simulink model "IGRF_Model"  (R2024a)
settings: Solver=VariableStepAuto  StartTime=0.0  StopTime=10.0  RelTol=1e-3
undefined symbols (not defined in the file or in its folder): WMM2020
libraries: sharedtransform x1, aerolibgravity2 x1
settings Model: Creator=hendr  LastModifiedBy=hendr

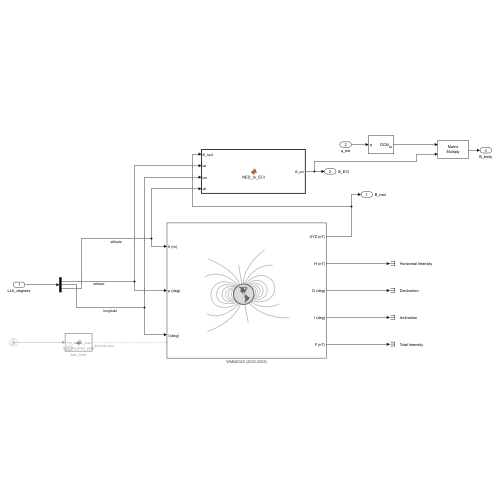
[thumbnail: Simulink's stored preview of the top-level diagram]
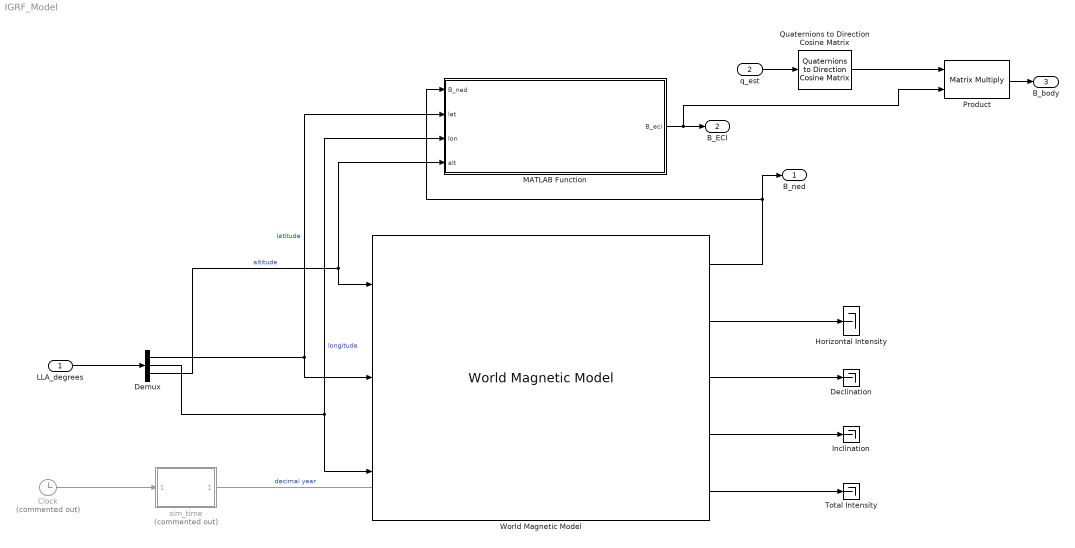
== system IGRF_Model ==
  LLA_degrees : Inport
  q_est : Inport  Port=2
  Clock : Clock  Commented=on
  Declination : Terminator
  Demux : Demux  Outputs=3
  Horizontal Intensity : Terminator
  Inclination : Terminator
  MATLAB Function : MATLAB Function  TreatAsAtomicUnit=on
  Product : Product  Multiplication=Matrix(*)
  Quaternions to Direction Cosine Matrix : sharedtransform/Quaternions to  Direction Cosine Matrix  aMode=aMode
      settings: LibrarySourceBlock=|
      | aerolibtransform2/Quaternions to
      | Direction Cosine Matrix
  Total Intensity : Terminator
  World Magnetic Model : aerolibgravity2/World Magnetic Model  model=WMM2020 (2020-2025)  customFile='WMM2020.COF'  units=Metric (MKS)  time_in=off  month=January  day=1  year=2020  action=Error  h_out=on  dec_out=on  inc_out=on  ti_out=on
  sim_time : MATLAB Function  Commented=on  TreatAsAtomicUnit=on
  B_ned : Outport
  B_ECI : Outport  Port=2
  B_body : Outport  Port=3
  wires:
  LLA_degrees/1 -> Demux/1
  Demux/1 -> MATLAB Function/2(lat), World Magnetic Model/2  "latitude"
  Demux/3 -> World Magnetic Model/1, MATLAB Function/4(alt)  "altitude"
  Demux/2 -> World Magnetic Model/3, MATLAB Function/3(lon)  "longitude"
  Clock/1 -> sim_time/1(sim_time)
  sim_time/1(dec_year) -> ?  "decimal year"
  World Magnetic Model/3 -> Declination/1
  World Magnetic Model/2 -> Horizontal Intensity/1
  World Magnetic Model/5 -> Total Intensity/1
  World Magnetic Model/4 -> Inclination/1
  World Magnetic Model/1 -> MATLAB Function/1(B_ned), B_ned/1
  MATLAB Function/1(B_eci) -> Product/2, B_ECI/1
  Quaternions to Direction Cosine Matrix/1 -> Product/1
  q_est/1 -> Quaternions to Direction Cosine Matrix/1
  Product/1 -> B_body/1

== matlab function IGRF_Model/sim_time ==
  data: sim_time input; dec_year output
function dec_year = get_decimal_year(sim_time)
% Convert simulation time (seconds) to decimal year
    base_year = 2026.0;                    % Update to current year
    seconds_per_year = 365.25 * 86400;    % Approximate
    dec_year = base_year + (sim_time / seconds_per_year);
end

== matlab function IGRF_Model/MATLAB Function ==
  data: B_ned input; B_eci output; lat input; lon input; alt input
function B_eci = NED_to_ECI(B_ned, lat, lon, alt)
% B_ned: Magnetic field in NED [North; East; Down] (Tesla)
% lat, lon in degrees, alt in meters

% Rotation matrix from NED to ECEF
R_ned2ecef = [ -sind(lat)*cosd(lon), -sind(lon), -cosd(lat)*cosd(lon);
               -sind(lat)*sind(lon),  cosd(lon), -cosd(lat)*sind(lon);
                cosd(lat),            0,        -sind(lat) ];

B_ecef = R_ned2ecef * B_ned;

% Convert ECEF to ECI (simple rotation using Greenwich Sidereal Time)
% For most AOCS simulations, you can approximate or use full transformation
% Use Aerospace Toolbox function if available
B_eci = B_ecef;  % Placeholder - replace with full ECEF->ECI if needed

end
